simulink model "Question_5"  (R2021a)
settings: Solver=VariableStepAuto  StartTime=0.0  StopTime=10.0  RelTol=1e-3
settings Model: Creator=haden  LastModifiedBy=haden

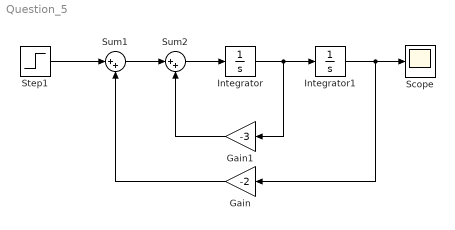
== system Question_5 ==
  Gain : Gain  Gain=-2
  Gain1 : Gain  Gain=-3
  Integrator : Integrator
  Integrator1 : Integrator
  Scope : Scope
  Step1 : Step  Time=0  SampleTime=0
  Sum1 : Sum  Inputs=|++
  Sum2 : Sum  Inputs=|++
  wires:
  Integrator/1 -> Gain1/1, Integrator1/1
  Gain/1 -> Sum1/2
  Integrator1/1 -> Scope/1, Gain/1
  Gain1/1 -> Sum2/2
  Sum2/1 -> Integrator/1
  Sum1/1 -> Sum2/1
  Step1/1 -> Sum1/1
